simulink model "MVDR_example_hdl_4x4_systolic"  (R2020a)
settings: Solver=FixedStepDiscrete  StartTime=0.0  StopTime=stoptime  RelTol=1e-3
InitFcn:
  | model_init
values from neighbouring files (symbols this model uses):
  BackSubstitutePrototype = fi(0, matrixdivbacksub_dt)    [model_init.m]
  matrixDivDelay = NumberOfCORDICIterations*10 + 86    [model_init.m]
  movavg_bitshift = nextpow2(sqrt(windowSize))    [model_init.m]
  mvdrPipelineDelay = covMatDelay+movAvgDelay+matrixDivDelay+normResponseDelay    [model_init.m]
  numArrayElements = 4    [model_init.m]
  NumberOfCORDICIterations = matrixdivin_dt.WordLength - 1    [model_init.m]
  srcAngles = [20 60]    [model_init.m]
  sv = step(steeringVector,fc,[scanAngle; 0])    [model_init.m]
  Ts = 1/fs    (= 7.8125e-09)    [model_init.m]
  windowSize = 1024    [model_init.m]
libraries: hdlsllib x249, simulink x44, commfilt2 x4, commrfcorlib x3, commsync2 x3, commrflib2 x2, commrandsrc3 x2, phasedtxrxlib x2, commdigbbndcpm2 x1, dspsolvers x1, embreciprocals x1, commdigbbndpm3 x1
(part 4 of 11)

== system MVDR_example_hdl_4x4_systolic/MVDR HDL/Compute Weight Vector/Matrix Left Divide/CORDIC/4x4 Complex CORDIC Matrix Left Divide/Back Substitute 4x4 Complex CORDIC/Invert first element - Folded1/ValidIn to Ready Logic ==
  readyIn : Inport
  validIn : Inport  Port=2
  AND : Logic  IconShape=distinctive  AllPortsSameDT=off  OutDataTypeStr=boolean
  NOT : Logic  Operator=NOT  IconShape=distinctive  AllPortsSameDT=off  OutDataTypeStr=boolean
  readyOut : Outport  VectorParamsAs1DForOutWhenUnconnected=off
  wires:
  validIn/1 -> NOT/1
  readyIn/1 -> AND/1
  AND/1 -> readyOut/1
  NOT/1 -> AND/2

== system MVDR_example_hdl_4x4_systolic/MVDR HDL/Compute Weight Vector/Matrix Left Divide/CORDIC/4x4 Complex CORDIC Matrix Left Divide/Back Substitute 4x4 Complex CORDIC/Invert first element - Folded2/CORDIC Reciprocal Normalized, Folded ==
  x : Inport
  validIn : Inport  Port=2
  CORDIC Reciprocal Rotations- Folded : Subsystem  TreatAsAtomicUnit=on  mask{NumberOfCORDICIterations=NumberOfCORDICIterations}
      mask prompts: NumberOfCORDICIterations "Number of CORDIC Iterations"
  Change sign : MATLAB Function  TreatAsAtomicUnit=on
  Delay{,1..3,5,10} (6 alike) : Delay  DelayLength=1
  Normalizer : Subsystem
  State Control : StateControl  StateControl=Synchronous
  Unit Delay Enabled Synchronous : hdlsllib/Discrete/Unit Delay Enabled Synchronous  InitialCondition=0.0  SampleTime=-1
      settings: SourceProductBaseCode=SL
  Unit Delay Enabled Synchronous1 : hdlsllib/Discrete/Unit Delay Enabled Synchronous  InitialCondition=0.0  SampleTime=-1
      settings: SourceProductBaseCode=SL
  ValidIn to Ready Logic : Subsystem
  ValidIn to Ready Logic1 : Subsystem
  ValidIn to Ready Logic2 : Subsystem
  1/x_normalized : Outport  VectorParamsAs1DForOutWhenUnconnected=off
  shift_value : Outport  Port=2  VectorParamsAs1DForOutWhenUnconnected=off
  validOut : Outport  Port=3  VectorParamsAs1DForOutWhenUnconnected=off
  ready : Outport  Port=4  VectorParamsAs1DForOutWhenUnconnected=off
  wires:
  Delay1/1 -> ValidIn to Ready Logic/2(validIn), CORDIC Reciprocal Rotations- Folded/2(validIn)
  Delay2/1 -> validOut/1
  CORDIC Reciprocal Rotations- Folded/2(validOut) -> Delay2/1
  ValidIn to Ready Logic2/1(readyOut) -> ready/1
  ValidIn to Ready Logic1/1(readyOut) -> ValidIn to Ready Logic2/1(readyIn)
  ValidIn to Ready Logic/1(readyOut) -> ValidIn to Ready Logic1/1(readyIn)
  CORDIC Reciprocal Rotations- Folded/3(ready) -> ValidIn to Ready Logic/1(readyIn)
  Delay10/1 -> Normalizer/2(validIn), ValidIn to Ready Logic2/2(validIn)
  validIn/1 -> Delay10/1, Unit Delay Enabled Synchronous/2
  Normalizer/4(validOut) -> Unit Delay Enabled Synchronous1/2, Delay1/1, ValidIn to Ready Logic1/2(validIn)
  Delay/1 -> CORDIC Reciprocal Rotations- Folded/1(x_in)
  x/1 -> Unit Delay Enabled Synchronous/1
  Normalizer/3(shift_amount) -> Unit Delay Enabled Synchronous1/1
  CORDIC Reciprocal Rotations- Folded/1(z_out) -> Change sign/1(x)
  Delay5/1 -> shift_value/1
  Normalizer/2(is_negative) -> Change sign/2(is_negative)
  Delay3/1 -> 1/x_normalized/1
  Unit Delay Enabled Synchronous1/1 -> Delay5/1
  Change sign/1(y) -> Delay3/1
  Normalizer/1(u_normalized) -> Delay/1
  Unit Delay Enabled Synchronous/1 -> Normalizer/1(u)

== system MVDR_example_hdl_4x4_systolic/MVDR HDL/Compute Weight Vector/Matrix Left Divide/CORDIC/4x4 Complex CORDIC Matrix Left Divide/Back Substitute 4x4 Complex CORDIC/Invert first element - Folded2/ValidIn to Ready Logic ==
  readyIn : Inport
  validIn : Inport  Port=2
  AND : Logic  IconShape=distinctive  AllPortsSameDT=off  OutDataTypeStr=boolean
  NOT : Logic  Operator=NOT  IconShape=distinctive  AllPortsSameDT=off  OutDataTypeStr=boolean
  readyOut : Outport  VectorParamsAs1DForOutWhenUnconnected=off
  wires:
  validIn/1 -> NOT/1
  readyIn/1 -> AND/1
  AND/1 -> readyOut/1
  NOT/1 -> AND/2

== system MVDR_example_hdl_4x4_systolic/MVDR HDL/Compute Weight Vector/Matrix Left Divide/CORDIC/4x4 Complex CORDIC Matrix Left Divide/Back Substitute 4x4 Complex CORDIC/Invert first element - Folded3/CORDIC Reciprocal Normalized, Folded ==
  x : Inport
  validIn : Inport  Port=2
  CORDIC Reciprocal Rotations- Folded : Subsystem  TreatAsAtomicUnit=on  mask{NumberOfCORDICIterations=NumberOfCORDICIterations}
      mask prompts: NumberOfCORDICIterations "Number of CORDIC Iterations"
  Change sign : MATLAB Function  TreatAsAtomicUnit=on
  Delay{,1..3,5,10} (6 alike) : Delay  DelayLength=1
  Normalizer : Subsystem
  State Control : StateControl  StateControl=Synchronous
  Unit Delay Enabled Synchronous : hdlsllib/Discrete/Unit Delay Enabled Synchronous  InitialCondition=0.0  SampleTime=-1
      settings: SourceProductBaseCode=SL
  Unit Delay Enabled Synchronous1 : hdlsllib/Discrete/Unit Delay Enabled Synchronous  InitialCondition=0.0  SampleTime=-1
      settings: SourceProductBaseCode=SL
  ValidIn to Ready Logic : Subsystem
  ValidIn to Ready Logic1 : Subsystem
  ValidIn to Ready Logic2 : Subsystem
  1/x_normalized : Outport  VectorParamsAs1DForOutWhenUnconnected=off
  shift_value : Outport  Port=2  VectorParamsAs1DForOutWhenUnconnected=off
  validOut : Outport  Port=3  VectorParamsAs1DForOutWhenUnconnected=off
  ready : Outport  Port=4  VectorParamsAs1DForOutWhenUnconnected=off
  wires:
  Delay1/1 -> ValidIn to Ready Logic/2(validIn), CORDIC Reciprocal Rotations- Folded/2(validIn)
  Delay2/1 -> validOut/1
  CORDIC Reciprocal Rotations- Folded/2(validOut) -> Delay2/1
  ValidIn to Ready Logic2/1(readyOut) -> ready/1
  ValidIn to Ready Logic1/1(readyOut) -> ValidIn to Ready Logic2/1(readyIn)
  ValidIn to Ready Logic/1(readyOut) -> ValidIn to Ready Logic1/1(readyIn)
  CORDIC Reciprocal Rotations- Folded/3(ready) -> ValidIn to Ready Logic/1(readyIn)
  Delay10/1 -> Normalizer/2(validIn), ValidIn to Ready Logic2/2(validIn)
  validIn/1 -> Delay10/1, Unit Delay Enabled Synchronous/2
  Normalizer/4(validOut) -> Unit Delay Enabled Synchronous1/2, Delay1/1, ValidIn to Ready Logic1/2(validIn)
  Delay/1 -> CORDIC Reciprocal Rotations- Folded/1(x_in)
  x/1 -> Unit Delay Enabled Synchronous/1
  Normalizer/3(shift_amount) -> Unit Delay Enabled Synchronous1/1
  CORDIC Reciprocal Rotations- Folded/1(z_out) -> Change sign/1(x)
  Delay5/1 -> shift_value/1
  Normalizer/2(is_negative) -> Change sign/2(is_negative)
  Delay3/1 -> 1/x_normalized/1
  Unit Delay Enabled Synchronous1/1 -> Delay5/1
  Change sign/1(y) -> Delay3/1
  Normalizer/1(u_normalized) -> Delay/1
  Unit Delay Enabled Synchronous/1 -> Normalizer/1(u)

== system MVDR_example_hdl_4x4_systolic/MVDR HDL/Compute Weight Vector/Matrix Left Divide/CORDIC/4x4 Complex CORDIC Matrix Left Divide/Back Substitute 4x4 Complex CORDIC/Invert first element - Folded3/ValidIn to Ready Logic ==
  readyIn : Inport
  validIn : Inport  Port=2
  AND : Logic  IconShape=distinctive  AllPortsSameDT=off  OutDataTypeStr=boolean
  NOT : Logic  Operator=NOT  IconShape=distinctive  AllPortsSameDT=off  OutDataTypeStr=boolean
  readyOut : Outport  VectorParamsAs1DForOutWhenUnconnected=off
  wires:
  validIn/1 -> NOT/1
  readyIn/1 -> AND/1
  AND/1 -> readyOut/1
  NOT/1 -> AND/2

== system MVDR_example_hdl_4x4_systolic/MVDR HDL/Compute Weight Vector/Matrix Left Divide/CORDIC/4x4 Complex CORDIC Matrix Left Divide/Back Substitute 4x4 Complex CORDIC/Row1 Back Substitute Specify Output Type/Cast like prototype ==
  In1 : Inport
  Cast like output prototype : MATLAB Function  TreatAsAtomicUnit=on
  Out1 : Outport  VectorParamsAs1DForOutWhenUnconnected=off
  wires:
  In1/1 -> Cast like output prototype/1(x)
  Cast like output prototype/1(y) -> Out1/1

== system MVDR_example_hdl_4x4_systolic/MVDR HDL/Compute Weight Vector/Matrix Left Divide/CORDIC/4x4 Complex CORDIC Matrix Left Divide/Back Substitute 4x4 Complex CORDIC/Row1 Back Substitute Specify Output Type/Variable shift ==
  x : Inport
  shift_value : Inport  Port=2
  MATLAB Function : MATLAB Function  TreatAsAtomicUnit=on
  y : Outport  VectorParamsAs1DForOutWhenUnconnected=off
  wires:
  shift_value/1 -> MATLAB Function/2(shift_value)
  MATLAB Function/1(y) -> y/1
  x/1 -> MATLAB Function/1(x)

== system MVDR_example_hdl_4x4_systolic/MVDR HDL/Compute Weight Vector/Matrix Left Divide/CORDIC/4x4 Complex CORDIC Matrix Left Divide/Back Substitute 4x4 Complex CORDIC/Row1 Back Substitute Specify Output Type/x2*r1(2) ==
  note: Xilinx devices:
      | - Set D1 = 1-2, D4 = 1, D5 = 1
      | - Use sync reset
      |
      | Intel FPGAs:
      | - Set D1 = 1, D4 = 0, D5 = 1
      | - Use async reset
  In1 : Inport
  In2 : Inport  Port=2
  Add1 : Sum  Inputs=+-
  Add2 : Sum
  Complex to Real-Imag : ComplexToRealImag
  Complex to Real-Imag1 : ComplexToRealImag
  D1_1 : Delay  DelayLength=1
  D1_2 : Delay  DelayLength=1
  D4_{1..4} (4 alike) : Delay  DelayLength=1
  D5_1 : Delay  DelayLength=1
  D5_2 : Delay  DelayLength=1
  Product{1..4} (4 alike) : Product  OutDataTypeStr=Inherit: Same as first input
  Real-Imag to Complex : RealImagToComplex
  Out1 : Outport  VectorParamsAs1DForOutWhenUnconnected=off
  wires:
  D4_4/1 -> Add2/2
  D4_2/1 -> Add1/2
  Product4/1 -> D4_4/1
  D4_3/1 -> Add2/1
  Product2/1 -> D4_2/1
  D4_1/1 -> Add1/1
  D5_2/1 -> Real-Imag to Complex/2
  D5_1/1 -> Real-Imag to Complex/1
  Add2/1 -> D5_2/1
  Add1/1 -> D5_1/1
  Product3/1 -> D4_3/1
  Product1/1 -> D4_1/1
  Complex to Real-Imag1/2 -> Product2/2, Product4/2  "D"
  Complex to Real-Imag/2 -> Product2/1, Product3/1  "B"
  Complex to Real-Imag1/1 -> Product1/2, Product3/2  "C"
  Complex to Real-Imag/1 -> Product1/1, Product4/1  "A"
  D1_2/1 -> Complex to Real-Imag1/1
  D1_1/1 -> Complex to Real-Imag/1
  Real-Imag to Complex/1 -> Out1/1
  In1/1 -> D1_1/1
  In2/1 -> D1_2/1

== system MVDR_example_hdl_4x4_systolic/MVDR HDL/Compute Weight Vector/Matrix Left Divide/CORDIC/4x4 Complex CORDIC Matrix Left Divide/Back Substitute 4x4 Complex CORDIC/Row1 Back Substitute Specify Output Type/x3*r1(3) ==
  note: Xilinx devices:
      | - Set D1 = 1-2, D4 = 1, D5 = 1
      | - Use sync reset
      |
      | Intel FPGAs:
      | - Set D1 = 1, D4 = 0, D5 = 1
      | - Use async reset
  In1 : Inport
  In2 : Inport  Port=2
  Add1 : Sum  Inputs=+-
  Add2 : Sum
  Complex to Real-Imag : ComplexToRealImag
  Complex to Real-Imag1 : ComplexToRealImag
  D1_1 : Delay  DelayLength=1
  D1_2 : Delay  DelayLength=1
  D4_{1..4} (4 alike) : Delay  DelayLength=1
  D5_1 : Delay  DelayLength=1
  D5_2 : Delay  DelayLength=1
  Product{1..4} (4 alike) : Product  OutDataTypeStr=Inherit: Same as first input
  Real-Imag to Complex : RealImagToComplex
  Out1 : Outport  VectorParamsAs1DForOutWhenUnconnected=off
  wires:
  D4_4/1 -> Add2/2
  D4_2/1 -> Add1/2
  Product4/1 -> D4_4/1
  D4_3/1 -> Add2/1
  Product2/1 -> D4_2/1
  D4_1/1 -> Add1/1
  D5_2/1 -> Real-Imag to Complex/2
  D5_1/1 -> Real-Imag to Complex/1
  Add2/1 -> D5_2/1
  Add1/1 -> D5_1/1
  Product3/1 -> D4_3/1
  Product1/1 -> D4_1/1
  Complex to Real-Imag1/2 -> Product2/2, Product4/2  "D"
  Complex to Real-Imag/2 -> Product2/1, Product3/1  "B"
  Complex to Real-Imag1/1 -> Product1/2, Product3/2  "C"
  Complex to Real-Imag/1 -> Product1/1, Product4/1  "A"
  D1_2/1 -> Complex to Real-Imag1/1
  D1_1/1 -> Complex to Real-Imag/1
  Real-Imag to Complex/1 -> Out1/1
  In1/1 -> D1_1/1
  In2/1 -> D1_2/1

== system MVDR_example_hdl_4x4_systolic/MVDR HDL/Compute Weight Vector/Matrix Left Divide/CORDIC/4x4 Complex CORDIC Matrix Left Divide/Back Substitute 4x4 Complex CORDIC/Row1 Back Substitute Specify Output Type/x4*r1(4) ==
  note: Xilinx devices:
      | - Set D1 = 1-2, D4 = 1, D5 = 1
      | - Use sync reset
      |
      | Intel FPGAs:
      | - Set D1 = 1, D4 = 0, D5 = 1
      | - Use async reset
  In1 : Inport
  In2 : Inport  Port=2
  Add1 : Sum  Inputs=+-
  Add2 : Sum
  Complex to Real-Imag : ComplexToRealImag
  Complex to Real-Imag1 : ComplexToRealImag
  D1_1 : Delay  DelayLength=1
  D1_2 : Delay  DelayLength=1
  D4_{1..4} (4 alike) : Delay  DelayLength=1
  D5_1 : Delay  DelayLength=1
  D5_2 : Delay  DelayLength=1
  Product{1..4} (4 alike) : Product  OutDataTypeStr=Inherit: Same as first input
  Real-Imag to Complex : RealImagToComplex
  Out1 : Outport  VectorParamsAs1DForOutWhenUnconnected=off
  wires:
  D4_4/1 -> Add2/2
  D4_2/1 -> Add1/2
  Product4/1 -> D4_4/1
  D4_3/1 -> Add2/1
  Product2/1 -> D4_2/1
  D4_1/1 -> Add1/1
  D5_2/1 -> Real-Imag to Complex/2
  D5_1/1 -> Real-Imag to Complex/1
  Add2/1 -> D5_2/1
  Add1/1 -> D5_1/1
  Product3/1 -> D4_3/1
  Product1/1 -> D4_1/1
  Complex to Real-Imag1/2 -> Product2/2, Product4/2  "D"
  Complex to Real-Imag/2 -> Product2/1, Product3/1  "B"
  Complex to Real-Imag1/1 -> Product1/2, Product3/2  "C"
  Complex to Real-Imag/1 -> Product1/1, Product4/1  "A"
  D1_2/1 -> Complex to Real-Imag1/1
  D1_1/1 -> Complex to Real-Imag/1
  Real-Imag to Complex/1 -> Out1/1
  In1/1 -> D1_1/1
  In2/1 -> D1_2/1

== system MVDR_example_hdl_4x4_systolic/MVDR HDL/Compute Weight Vector/Matrix Left Divide/CORDIC/4x4 Complex CORDIC Matrix Left Divide/Back Substitute 4x4 Complex CORDIC/Row2 Back Substitute Specify Output Type/Cast like prototype ==
  In1 : Inport
  Cast like output prototype : MATLAB Function  TreatAsAtomicUnit=on
  Out1 : Outport  VectorParamsAs1DForOutWhenUnconnected=off
  wires:
  In1/1 -> Cast like output prototype/1(x)
  Cast like output prototype/1(y) -> Out1/1

== system MVDR_example_hdl_4x4_systolic/MVDR HDL/Compute Weight Vector/Matrix Left Divide/CORDIC/4x4 Complex CORDIC Matrix Left Divide/Back Substitute 4x4 Complex CORDIC/Row2 Back Substitute Specify Output Type/Variable shift ==
  x : Inport
  shift_value : Inport  Port=2
  MATLAB Function : MATLAB Function  TreatAsAtomicUnit=on
  y : Outport  VectorParamsAs1DForOutWhenUnconnected=off
  wires:
  shift_value/1 -> MATLAB Function/2(shift_value)
  MATLAB Function/1(y) -> y/1
  x/1 -> MATLAB Function/1(x)

== system MVDR_example_hdl_4x4_systolic/MVDR HDL/Compute Weight Vector/Matrix Left Divide/CORDIC/4x4 Complex CORDIC Matrix Left Divide/Back Substitute 4x4 Complex CORDIC/Row2 Back Substitute Specify Output Type/x3*r2(2) ==
  note: Xilinx devices:
      | - Set D1 = 1-2, D4 = 1, D5 = 1
      | - Use sync reset
      |
      | Intel FPGAs:
      | - Set D1 = 1, D4 = 0, D5 = 1
      | - Use async reset
  In1 : Inport
  In2 : Inport  Port=2
  Add1 : Sum  Inputs=+-
  Add2 : Sum
  Complex to Real-Imag : ComplexToRealImag
  Complex to Real-Imag1 : ComplexToRealImag
  D1_1 : Delay  DelayLength=1
  D1_2 : Delay  DelayLength=1
  D4_{1..4} (4 alike) : Delay  DelayLength=1
  D5_1 : Delay  DelayLength=1
  D5_2 : Delay  DelayLength=1
  Product{1..4} (4 alike) : Product  OutDataTypeStr=Inherit: Same as first input
  Real-Imag to Complex : RealImagToComplex
  Out1 : Outport  VectorParamsAs1DForOutWhenUnconnected=off
  wires:
  D4_4/1 -> Add2/2
  D4_2/1 -> Add1/2
  Product4/1 -> D4_4/1
  D4_3/1 -> Add2/1
  Product2/1 -> D4_2/1
  D4_1/1 -> Add1/1
  D5_2/1 -> Real-Imag to Complex/2
  D5_1/1 -> Real-Imag to Complex/1
  Add2/1 -> D5_2/1
  Add1/1 -> D5_1/1
  Product3/1 -> D4_3/1
  Product1/1 -> D4_1/1
  Complex to Real-Imag1/2 -> Product2/2, Product4/2  "D"
  Complex to Real-Imag/2 -> Product2/1, Product3/1  "B"
  Complex to Real-Imag1/1 -> Product1/2, Product3/2  "C"
  Complex to Real-Imag/1 -> Product1/1, Product4/1  "A"
  D1_2/1 -> Complex to Real-Imag1/1
  D1_1/1 -> Complex to Real-Imag/1
  Real-Imag to Complex/1 -> Out1/1
  In1/1 -> D1_1/1
  In2/1 -> D1_2/1

== system MVDR_example_hdl_4x4_systolic/MVDR HDL/Compute Weight Vector/Matrix Left Divide/CORDIC/4x4 Complex CORDIC Matrix Left Divide/Back Substitute 4x4 Complex CORDIC/Row2 Back Substitute Specify Output Type/x4*r2(3) ==
  note: Xilinx devices:
      | - Set D1 = 1-2, D4 = 1, D5 = 1
      | - Use sync reset
      |
      | Intel FPGAs:
      | - Set D1 = 1, D4 = 0, D5 = 1
      | - Use async reset
  In1 : Inport
  In2 : Inport  Port=2
  Add1 : Sum  Inputs=+-
  Add2 : Sum
  Complex to Real-Imag : ComplexToRealImag
  Complex to Real-Imag1 : ComplexToRealImag
  D1_1 : Delay  DelayLength=1
  D1_2 : Delay  DelayLength=1
  D4_{1..4} (4 alike) : Delay  DelayLength=1
  D5_1 : Delay  DelayLength=1
  D5_2 : Delay  DelayLength=1
  Product{1..4} (4 alike) : Product  OutDataTypeStr=Inherit: Same as first input
  Real-Imag to Complex : RealImagToComplex
  Out1 : Outport  VectorParamsAs1DForOutWhenUnconnected=off
  wires:
  D4_4/1 -> Add2/2
  D4_2/1 -> Add1/2
  Product4/1 -> D4_4/1
  D4_3/1 -> Add2/1
  Product2/1 -> D4_2/1
  D4_1/1 -> Add1/1
  D5_2/1 -> Real-Imag to Complex/2
  D5_1/1 -> Real-Imag to Complex/1
  Add2/1 -> D5_2/1
  Add1/1 -> D5_1/1
  Product3/1 -> D4_3/1
  Product1/1 -> D4_1/1
  Complex to Real-Imag1/2 -> Product2/2, Product4/2  "D"
  Complex to Real-Imag/2 -> Product2/1, Product3/1  "B"
  Complex to Real-Imag1/1 -> Product1/2, Product3/2  "C"
  Complex to Real-Imag/1 -> Product1/1, Product4/1  "A"
  D1_2/1 -> Complex to Real-Imag1/1
  D1_1/1 -> Complex to Real-Imag/1
  Real-Imag to Complex/1 -> Out1/1
  In1/1 -> D1_1/1
  In2/1 -> D1_2/1

== system MVDR_example_hdl_4x4_systolic/MVDR HDL/Compute Weight Vector/Matrix Left Divide/CORDIC/4x4 Complex CORDIC Matrix Left Divide/Back Substitute 4x4 Complex CORDIC/Row3 Back Substitute Specify Output Type/Cast like prototype ==
  In1 : Inport
  Cast like output prototype : MATLAB Function  TreatAsAtomicUnit=on
  Out1 : Outport  VectorParamsAs1DForOutWhenUnconnected=off
  wires:
  In1/1 -> Cast like output prototype/1(x)
  Cast like output prototype/1(y) -> Out1/1

== system MVDR_example_hdl_4x4_systolic/MVDR HDL/Compute Weight Vector/Matrix Left Divide/CORDIC/4x4 Complex CORDIC Matrix Left Divide/Back Substitute 4x4 Complex CORDIC/Row3 Back Substitute Specify Output Type/Cast like prototype1 ==
  In1 : Inport
  Cast like output prototype : MATLAB Function  TreatAsAtomicUnit=on
  Out1 : Outport  VectorParamsAs1DForOutWhenUnconnected=off
  wires:
  In1/1 -> Cast like output prototype/1(x)
  Cast like output prototype/1(y) -> Out1/1

== system MVDR_example_hdl_4x4_systolic/MVDR HDL/Compute Weight Vector/Matrix Left Divide/CORDIC/4x4 Complex CORDIC Matrix Left Divide/Back Substitute 4x4 Complex CORDIC/Row3 Back Substitute Specify Output Type/Variable shift ==
  x : Inport
  shift_value : Inport  Port=2
  MATLAB Function : MATLAB Function  TreatAsAtomicUnit=on
  y : Outport  VectorParamsAs1DForOutWhenUnconnected=off
  wires:
  shift_value/1 -> MATLAB Function/2(shift_value)
  MATLAB Function/1(y) -> y/1
  x/1 -> MATLAB Function/1(x)

== system MVDR_example_hdl_4x4_systolic/MVDR HDL/Compute Weight Vector/Matrix Left Divide/CORDIC/4x4 Complex CORDIC Matrix Left Divide/Back Substitute 4x4 Complex CORDIC/Row3 Back Substitute Specify Output Type/r3(2)*x4 ==
  note: Xilinx devices:
      | - Set D1 = 1-2, D4 = 1, D5 = 1
      | - Use sync reset
      |
      | Intel FPGAs:
      | - Set D1 = 1, D4 = 0, D5 = 1
      | - Use async reset
  In1 : Inport
  In2 : Inport  Port=2
  Add1 : Sum  Inputs=+-
  Add2 : Sum
  Complex to Real-Imag : ComplexToRealImag
  Complex to Real-Imag1 : ComplexToRealImag
  D1_1 : Delay  DelayLength=1
  D1_2 : Delay  DelayLength=1
  D4_{1..4} (4 alike) : Delay  DelayLength=1
  D5_1 : Delay  DelayLength=1
  D5_2 : Delay  DelayLength=1
  Product{1..4} (4 alike) : Product  OutDataTypeStr=Inherit: Same as first input
  Real-Imag to Complex : RealImagToComplex
  Out1 : Outport  VectorParamsAs1DForOutWhenUnconnected=off
  wires:
  D4_4/1 -> Add2/2
  D4_2/1 -> Add1/2
  Product4/1 -> D4_4/1
  D4_3/1 -> Add2/1
  Product2/1 -> D4_2/1
  D4_1/1 -> Add1/1
  D5_2/1 -> Real-Imag to Complex/2
  D5_1/1 -> Real-Imag to Complex/1
  Add2/1 -> D5_2/1
  Add1/1 -> D5_1/1
  Product3/1 -> D4_3/1
  Product1/1 -> D4_1/1
  Complex to Real-Imag1/2 -> Product2/2, Product4/2  "D"
  Complex to Real-Imag/2 -> Product2/1, Product3/1  "B"
  Complex to Real-Imag1/1 -> Product1/2, Product3/2  "C"
  Complex to Real-Imag/1 -> Product1/1, Product4/1  "A"
  D1_2/1 -> Complex to Real-Imag1/1
  D1_1/1 -> Complex to Real-Imag/1
  Real-Imag to Complex/1 -> Out1/1
  In1/1 -> D1_1/1
  In2/1 -> D1_2/1

== system MVDR_example_hdl_4x4_systolic/MVDR HDL/Compute Weight Vector/Matrix Left Divide/CORDIC/4x4 Complex CORDIC Matrix Left Divide/Back Substitute 4x4 Complex CORDIC/Row4 Back Substitute Specify Output Type/Cast like prototype ==
  In1 : Inport
  Cast like output prototype : MATLAB Function  TreatAsAtomicUnit=on
  Out1 : Outport  VectorParamsAs1DForOutWhenUnconnected=off
  wires:
  In1/1 -> Cast like output prototype/1(x)
  Cast like output prototype/1(y) -> Out1/1

== system MVDR_example_hdl_4x4_systolic/MVDR HDL/Compute Weight Vector/Matrix Left Divide/CORDIC/4x4 Complex CORDIC Matrix Left Divide/Back Substitute 4x4 Complex CORDIC/Row4 Back Substitute Specify Output Type/Variable shift ==
  x : Inport
  shift_value : Inport  Port=2
  MATLAB Function : MATLAB Function  TreatAsAtomicUnit=on
  y : Outport  VectorParamsAs1DForOutWhenUnconnected=off
  wires:
  shift_value/1 -> MATLAB Function/2(shift_value)
  MATLAB Function/1(y) -> y/1
  x/1 -> MATLAB Function/1(x)

== system MVDR_example_hdl_4x4_systolic/MVDR HDL/Compute Weight Vector/Matrix Left Divide/CORDIC/4x4 Complex CORDIC Matrix Left Divide/Q'B, R 4x4 Complex CORDIC Systolic Array/Complex Row Rotation with real pivots/Inverse CORDIC Gain1 ==
  In1 : Inport
  Inverse CORDIC Gain : Gain  Gain=1/prod(sqrt(1+2.^(-2*(0:double(NumberOfCORDICIterations)-1))))  OutDataTypeStr=Inherit: Same as input
  Out1 : Outport  VectorParamsAs1DForOutWhenUnconnected=off
  wires:
  Inverse CORDIC Gain/1 -> Out1/1
  In1/1 -> Inverse CORDIC Gain/1

== system MVDR_example_hdl_4x4_systolic/MVDR HDL/Compute Weight Vector/Matrix Left Divide/CORDIC/4x4 Complex CORDIC Matrix Left Divide/Q'B, R 4x4 Complex CORDIC Systolic Array/Complex Row Rotation with real pivots/Inverse CORDIC Gain2 ==
  In1 : Inport
  Inverse CORDIC Gain : Gain  Gain=1/prod(sqrt(1+2.^(-2*(0:double(NumberOfCORDICIterations)-1))))  OutDataTypeStr=Inherit: Same as input
  Out1 : Outport  VectorParamsAs1DForOutWhenUnconnected=off
  wires:
  Inverse CORDIC Gain/1 -> Out1/1
  In1/1 -> Inverse CORDIC Gain/1

== system MVDR_example_hdl_4x4_systolic/MVDR HDL/Compute Weight Vector/Matrix Left Divide/CORDIC/4x4 Complex CORDIC Matrix Left Divide/Q'B, R 4x4 Complex CORDIC Systolic Array/Complex Row Rotation with real pivots/Inverse CORDIC Gain3 ==
  In1 : Inport
  Inverse CORDIC Gain : Gain  Gain=1/prod(sqrt(1+2.^(-2*(0:double(NumberOfCORDICIterations)-1))))  OutDataTypeStr=Inherit: Same as input
  Out1 : Outport  VectorParamsAs1DForOutWhenUnconnected=off
  wires:
  Inverse CORDIC Gain/1 -> Out1/1
  In1/1 -> Inverse CORDIC Gain/1

== system MVDR_example_hdl_4x4_systolic/MVDR HDL/Compute Weight Vector/Matrix Left Divide/CORDIC/4x4 Complex CORDIC Matrix Left Divide/Q'B, R 4x4 Complex CORDIC Systolic Array/Complex Row Rotation with real pivots/Inverse CORDIC Gain4 ==
  In1 : Inport
  Inverse CORDIC Gain : Gain  Gain=1/prod(sqrt(1+2.^(-2*(0:double(NumberOfCORDICIterations)-1))))  OutDataTypeStr=Inherit: Same as input
  Out1 : Outport  VectorParamsAs1DForOutWhenUnconnected=off
  wires:
  Inverse CORDIC Gain/1 -> Out1/1
  In1/1 -> Inverse CORDIC Gain/1

== system MVDR_example_hdl_4x4_systolic/MVDR HDL/Compute Weight Vector/Matrix Left Divide/CORDIC/4x4 Complex CORDIC Matrix Left Divide/Q'B, R 4x4 Complex CORDIC Systolic Array/Complex Row Rotation with real pivots/Q'B, R Row Rotations - Complex ==
  x : Inport
  y : Inport  Port=2
  u : Inport  Port=3
  v : Inport  Port=4
  validIn : Inport  Port=5
  CORDIC Counter : Subsystem  mask{NumberOfCORDICIterations=NumberOfCORDICIterations}
      mask prompts: NumberOfCORDICIterations "Number of CORDIC Iterations"
  Delay{1..13} (13 alike) : Delay  DelayLength=1
  MATLAB Function : MATLAB Function  TreatAsAtomicUnit=on
  Same Datatype : Subsystem  TreatAsAtomicUnit=on
  Same Datatype1 : Subsystem  TreatAsAtomicUnit=on
  Same Datatype2 : Subsystem  TreatAsAtomicUnit=on
  Same Datatype3 : Subsystem  TreatAsAtomicUnit=on
  Switch{,1..3} (4 alike) : Switch  Criteria=u2 ~= 0
  x_out : Outport  VectorParamsAs1DForOutWhenUnconnected=off
  y_out : Outport  Port=2  VectorParamsAs1DForOutWhenUnconnected=off
  u_out : Outport  Port=3  VectorParamsAs1DForOutWhenUnconnected=off
  v_out : Outport  Port=4  VectorParamsAs1DForOutWhenUnconnected=off
  validOut : Outport  Port=5  VectorParamsAs1DForOutWhenUnconnected=off
  ready : Outport  Port=6  VectorParamsAs1DForOutWhenUnconnected=off
  wires:
  Delay13/1 -> ready/1
  Delay12/1 -> Delay3/1
  Delay10/1 -> MATLAB Function/5(iteration)
  Delay9/1 -> Switch3/2, Switch2/2, Switch1/2, Switch/2
  Delay8/1 -> Switch3/3, Same Datatype2/2(Reference)
  Delay6/1 -> Switch2/3, Same Datatype3/2(Reference)
  Delay5/1 -> Switch1/3, Same Datatype1/2(Reference)
  Delay4/1 -> Switch/3, Same Datatype/2(Reference)
  Same Datatype2/1(DataOut) -> Switch3/1
  Same Datatype3/1(DataOut) -> Switch2/1
  Same Datatype1/1(DataOut) -> Switch1/1
  Same Datatype/1(DataOut) -> Switch/1
  v/1 -> Delay8/1
  u/1 -> Delay6/1
  y/1 -> Delay5/1
  x/1 -> Delay4/1
  CORDIC Counter/1(count_is_positive) -> Delay9/1
  Switch3/1 -> MATLAB Function/4(v)
  Switch2/1 -> MATLAB Function/3(u)
  Switch1/1 -> MATLAB Function/2(y)
  Switch/1 -> MATLAB Function/1(x)
  CORDIC Counter/4(ready) -> Delay13/1
  CORDIC Counter/3(last) -> Delay12/1
  CORDIC Counter/2(count) -> Delay10/1
  validIn/1 -> CORDIC Counter/1(validIn)
  Delay3/1 -> validOut/1
  Delay7/1 -> u_out/1, Same Datatype3/1(Data)
  MATLAB Function/4(v_out) -> Delay11/1
  MATLAB Function/3(u_out) -> Delay7/1
  MATLAB Function/2(y_out) -> Delay2/1
  MATLAB Function/1(x_out) -> Delay1/1
  Delay11/1 -> v_out/1, Same Datatype2/1(Data)
  Delay2/1 -> y_out/1, Same Datatype1/1(Data)
  Delay1/1 -> x_out/1, Same Datatype/1(Data)

== system MVDR_example_hdl_4x4_systolic/MVDR HDL/Compute Weight Vector/Matrix Left Divide/CORDIC/4x4 Complex CORDIC Matrix Left Divide/Q'B, R 4x4 Complex CORDIC Systolic Array/Complex Row Rotation with real pivots/ValidIn to Ready Logic ==
  readyIn : Inport
  validIn : Inport  Port=2
  AND : Logic  IconShape=distinctive  AllPortsSameDT=off  OutDataTypeStr=boolean
  NOT : Logic  Operator=NOT  IconShape=distinctive  AllPortsSameDT=off  OutDataTypeStr=boolean
  readyOut : Outport  VectorParamsAs1DForOutWhenUnconnected=off
  wires:
  validIn/1 -> NOT/1
  readyIn/1 -> AND/1
  AND/1 -> readyOut/1
  NOT/1 -> AND/2

== system MVDR_example_hdl_4x4_systolic/MVDR HDL/Compute Weight Vector/Matrix Left Divide/CORDIC/4x4 Complex CORDIC Matrix Left Divide/Q'B, R 4x4 Complex CORDIC Systolic Array/Complex Row Rotation with real pivots/ValidIn to Ready Logic1 ==
  readyIn : Inport
  validIn : Inport  Port=2
  AND : Logic  IconShape=distinctive  AllPortsSameDT=off  OutDataTypeStr=boolean
  NOT : Logic  Operator=NOT  IconShape=distinctive  AllPortsSameDT=off  OutDataTypeStr=boolean
  readyOut : Outport  VectorParamsAs1DForOutWhenUnconnected=off
  wires:
  validIn/1 -> NOT/1
  readyIn/1 -> AND/1
  AND/1 -> readyOut/1
  NOT/1 -> AND/2

== system MVDR_example_hdl_4x4_systolic/MVDR HDL/Compute Weight Vector/Matrix Left Divide/CORDIC/4x4 Complex CORDIC Matrix Left Divide/Q'B, R 4x4 Complex CORDIC Systolic Array/Complex Row Rotation 1/Inverse CORDIC Gain1 ==
  In1 : Inport
  Inverse CORDIC Gain : Gain  Gain=1/prod(sqrt(1+2.^(-2*(0:double(NumberOfCORDICIterations)-1))))  OutDataTypeStr=Inherit: Same as input
  Out1 : Outport  VectorParamsAs1DForOutWhenUnconnected=off
  wires:
  Inverse CORDIC Gain/1 -> Out1/1
  In1/1 -> Inverse CORDIC Gain/1

== system MVDR_example_hdl_4x4_systolic/MVDR HDL/Compute Weight Vector/Matrix Left Divide/CORDIC/4x4 Complex CORDIC Matrix Left Divide/Q'B, R 4x4 Complex CORDIC Systolic Array/Complex Row Rotation 1/Inverse CORDIC Gain2 ==
  In1 : Inport
  Inverse CORDIC Gain : Gain  Gain=1/prod(sqrt(1+2.^(-2*(0:double(NumberOfCORDICIterations)-1))))  OutDataTypeStr=Inherit: Same as input
  Out1 : Outport  VectorParamsAs1DForOutWhenUnconnected=off
  wires:
  Inverse CORDIC Gain/1 -> Out1/1
  In1/1 -> Inverse CORDIC Gain/1

== system MVDR_example_hdl_4x4_systolic/MVDR HDL/Compute Weight Vector/Matrix Left Divide/CORDIC/4x4 Complex CORDIC Matrix Left Divide/Q'B, R 4x4 Complex CORDIC Systolic Array/Complex Row Rotation 1/Inverse CORDIC Gain3 ==
  In1 : Inport
  Inverse CORDIC Gain : Gain  Gain=1/prod(sqrt(1+2.^(-2*(0:double(NumberOfCORDICIterations)-1))))  OutDataTypeStr=Inherit: Same as input
  Out1 : Outport  VectorParamsAs1DForOutWhenUnconnected=off
  wires:
  Inverse CORDIC Gain/1 -> Out1/1
  In1/1 -> Inverse CORDIC Gain/1

== system MVDR_example_hdl_4x4_systolic/MVDR HDL/Compute Weight Vector/Matrix Left Divide/CORDIC/4x4 Complex CORDIC Matrix Left Divide/Q'B, R 4x4 Complex CORDIC Systolic Array/Complex Row Rotation 1/Inverse CORDIC Gain4 ==
  In1 : Inport
  Inverse CORDIC Gain : Gain  Gain=1/prod(sqrt(1+2.^(-2*(0:double(NumberOfCORDICIterations)-1))))  OutDataTypeStr=Inherit: Same as input
  Out1 : Outport  VectorParamsAs1DForOutWhenUnconnected=off
  wires:
  Inverse CORDIC Gain/1 -> Out1/1
  In1/1 -> Inverse CORDIC Gain/1

== system MVDR_example_hdl_4x4_systolic/MVDR HDL/Compute Weight Vector/Matrix Left Divide/CORDIC/4x4 Complex CORDIC Matrix Left Divide/Q'B, R 4x4 Complex CORDIC Systolic Array/Complex Row Rotation 1/Q'B, R Row Rotations - Complex - Folded ==
  x : Inport
  y : Inport  Port=2
  u : Inport  Port=3
  v : Inport  Port=4
  validIn : Inport  Port=5
  CORDIC Counter : Subsystem  mask{NumberOfCORDICIterations=NumberOfCORDICIterations}
      mask prompts: NumberOfCORDICIterations "Number of CORDIC Iterations"
  Delay{1..13} (13 alike) : Delay  DelayLength=1
  MATLAB Function : MATLAB Function  TreatAsAtomicUnit=on
  Same Datatype : Subsystem  TreatAsAtomicUnit=on
  Same Datatype1 : Subsystem  TreatAsAtomicUnit=on
  Same Datatype2 : Subsystem  TreatAsAtomicUnit=on
  Same Datatype3 : Subsystem  TreatAsAtomicUnit=on
  Switch{,1..3} (4 alike) : Switch  Criteria=u2 ~= 0
  x_out : Outport  VectorParamsAs1DForOutWhenUnconnected=off
  y_out : Outport  Port=2  VectorParamsAs1DForOutWhenUnconnected=off
  u_out : Outport  Port=3  VectorParamsAs1DForOutWhenUnconnected=off
  v_out : Outport  Port=4  VectorParamsAs1DForOutWhenUnconnected=off
  validOut : Outport  Port=5  VectorParamsAs1DForOutWhenUnconnected=off
  ready : Outport  Port=6  VectorParamsAs1DForOutWhenUnconnected=off
  wires:
  Delay13/1 -> ready/1
  Delay12/1 -> Delay3/1
  Delay10/1 -> MATLAB Function/5(iteration)
  Delay9/1 -> Switch3/2, Switch2/2, Switch1/2, Switch/2
  Delay8/1 -> Switch3/3, Same Datatype2/2(Reference)
  Delay6/1 -> Switch2/3, Same Datatype3/2(Reference)
  Delay5/1 -> Switch1/3, Same Datatype1/2(Reference)
  Delay4/1 -> Switch/3, Same Datatype/2(Reference)
  Same Datatype2/1(DataOut) -> Switch3/1
  Same Datatype3/1(DataOut) -> Switch2/1
  Same Datatype1/1(DataOut) -> Switch1/1
  Same Datatype/1(DataOut) -> Switch/1
  v/1 -> Delay8/1
  u/1 -> Delay6/1
  y/1 -> Delay5/1
  x/1 -> Delay4/1
  CORDIC Counter/1(count_is_positive) -> Delay9/1
  Switch3/1 -> MATLAB Function/4(v)
  Switch2/1 -> MATLAB Function/3(u)
  Switch1/1 -> MATLAB Function/2(y)
  Switch/1 -> MATLAB Function/1(x)
  CORDIC Counter/4(ready) -> Delay13/1
  CORDIC Counter/3(last) -> Delay12/1
  CORDIC Counter/2(count) -> Delay10/1
  validIn/1 -> CORDIC Counter/1(validIn)
  Delay3/1 -> validOut/1
  Delay7/1 -> u_out/1, Same Datatype3/1(Data)
  MATLAB Function/4(v_out) -> Delay11/1
  MATLAB Function/3(u_out) -> Delay7/1
  MATLAB Function/2(y_out) -> Delay2/1
  MATLAB Function/1(x_out) -> Delay1/1
  Delay11/1 -> v_out/1, Same Datatype2/1(Data)
  Delay2/1 -> y_out/1, Same Datatype1/1(Data)
  Delay1/1 -> x_out/1, Same Datatype/1(Data)

== system MVDR_example_hdl_4x4_systolic/MVDR HDL/Compute Weight Vector/Matrix Left Divide/CORDIC/4x4 Complex CORDIC Matrix Left Divide/Q'B, R 4x4 Complex CORDIC Systolic Array/Complex Row Rotation 1/Rotate first element to real - Folded ==
  x : Inport
  u : Inport  Port=2
  validIn : Inport  Port=3
  Complex to Real-Imag : ComplexToRealImag
  Complex to Real-Imag1 : ComplexToRealImag
  Delay{4..7,9..10,15} (7 alike) : Delay  DelayLength=1
  Force imaginary part to exactly zero : MATLAB Function  TreatAsAtomicUnit=on
  Inverse CORDIC Gain1 : Subsystem  TreatAsAtomicUnit=on  mask{NumberOfCORDICIterations=NumberOfCORDICIterations}
      mask prompts: NumberOfCORDICIterations "Number of CORDIC Iterations"
      mask Display: disp('1/An')
  Inverse CORDIC Gain2 : Subsystem  TreatAsAtomicUnit=on  mask{NumberOfCORDICIterations=NumberOfCORDICIterations}
      mask prompts: NumberOfCORDICIterations "Number of CORDIC Iterations"
      mask Display: disp('1/An')
  Inverse CORDIC Gain3 : Subsystem  TreatAsAtomicUnit=on  mask{NumberOfCORDICIterations=NumberOfCORDICIterations}
      mask prompts: NumberOfCORDICIterations "Number of CORDIC Iterations"
      mask Display: disp('1/An')
  Inverse CORDIC Gain4 : Subsystem  TreatAsAtomicUnit=on  mask{NumberOfCORDICIterations=NumberOfCORDICIterations}
      mask prompts: NumberOfCORDICIterations "Number of CORDIC Iterations"
      mask Display: disp('1/An')
  "Q'B, R Row Rotations - Real" : Subsystem  TreatAsAtomicUnit=on  mask{NumberOfCORDICIterations=NumberOfCORDICIterations}
      mask prompts: NumberOfCORDICIterations "Number of CORDIC Iterations"
  QR 3rd and 4th Quadrant Compensation : MATLAB Function  TreatAsAtomicUnit=on
  Real-Imag to Complex : RealImagToComplex
  Real-Imag to Complex1 : RealImagToComplex
  State Control : StateControl  StateControl=Synchronous
  Unit Delay Enabled Synchronous{,1..3} (4 alike) : hdlsllib/Discrete/Unit Delay Enabled Synchronous  InitialCondition=0.0  SampleTime=-1
      settings: SourceProductBaseCode=SL
  ValidIn to Ready Logic with Delay : Subsystem
  x' : Outport  VectorParamsAs1DForOutWhenUnconnected=off
  u' : Outport  Port=2  VectorParamsAs1DForOutWhenUnconnected=off
  validOut : Outport  Port=3  VectorParamsAs1DForOutWhenUnconnected=off
  ready : Outport  Port=4  VectorParamsAs1DForOutWhenUnconnected=off
  wires:
  Unit Delay Enabled Synchronous3/1 -> x'/1
  Real-Imag to Complex/1 -> Unit Delay Enabled Synchronous3/1
  Unit Delay Enabled Synchronous2/1 -> u'/1
  Real-Imag to Complex1/1 -> Unit Delay Enabled Synchronous2/1
  Unit Delay Enabled Synchronous1/1 -> Complex to Real-Imag/1
  Unit Delay Enabled Synchronous/1 -> Complex to Real-Imag1/1
  "Q'B, R Row Rotations - Real"/6(ready) -> ValidIn to Ready Logic with Delay/1(readyIn)
  ValidIn to Ready Logic with Delay/1(readyOut) -> ready/1
  Delay15/1 -> validOut/1
  "Q'B, R Row Rotations - Real"/5(validOut) -> Delay15/1, Unit Delay Enabled Synchronous3/2, Unit Delay Enabled Synchronous2/2
  Inverse CORDIC Gain3/1(Out1) -> Real-Imag to Complex1/2
  Inverse CORDIC Gain2/1(Out1) -> Real-Imag to Complex1/1
  Inverse CORDIC Gain1/1(Out1) -> Force imaginary part to exactly zero/1(u)
  Inverse CORDIC Gain4/1(Out1) -> Real-Imag to Complex/1
  Delay10/1 -> "Q'B, R Row Rotations - Real"/5(validIn), ValidIn to Ready Logic with Delay/2(validIn * z^-1)
  validIn/1 -> Delay9/1, Unit Delay Enabled Synchronous1/2, Unit Delay Enabled Synchronous/2
  Delay9/1 -> Delay10/1, ValidIn to Ready Logic with Delay/3(validIn)
  Force imaginary part to exactly zero/1(y) -> Real-Imag to Complex/2
  "Q'B, R Row Rotations - Real"/2(y_out) -> Inverse CORDIC Gain1/1(In1)
  u/1 -> Unit Delay Enabled Synchronous/1
  x/1 -> Unit Delay Enabled Synchronous1/1
  "Q'B, R Row Rotations - Real"/4(v_out) -> Inverse CORDIC Gain3/1(In1)
  "Q'B, R Row Rotations - Real"/3(u_out) -> Inverse CORDIC Gain2/1(In1)
  "Q'B, R Row Rotations - Real"/1(x_out) -> Inverse CORDIC Gain4/1(In1)
  Delay7/1 -> "Q'B, R Row Rotations - Real"/4(v)
  Delay6/1 -> "Q'B, R Row Rotations - Real"/3(u)
  Delay5/1 -> "Q'B, R Row Rotations - Real"/2(y)
  Delay4/1 -> "Q'B, R Row Rotations - Real"/1(x)
  Complex to Real-Imag1/2 -> QR 3rd and 4th Quadrant Compensation/4(v)
  Complex to Real-Imag1/1 -> QR 3rd and 4th Quadrant Compensation/3(u)
  Complex to Real-Imag/2 -> QR 3rd and 4th Quadrant Compensation/2(y)
  Complex to Real-Imag/1 -> QR 3rd and 4th Quadrant Compensation/1(x)
  QR 3rd and 4th Quadrant Compensation/4(v_out) -> Delay7/1
  QR 3rd and 4th Quadrant Compensation/2(y_out) -> Delay5/1
  QR 3rd and 4th Quadrant Compensation/3(u_out) -> Delay6/1
  QR 3rd and 4th Quadrant Compensation/1(x_out) -> Delay4/1

== system MVDR_example_hdl_4x4_systolic/MVDR HDL/Compute Weight Vector/Matrix Left Divide/CORDIC/4x4 Complex CORDIC Matrix Left Divide/Q'B, R 4x4 Complex CORDIC Systolic Array/Complex Row Rotation 1/ValidIn to Ready Logic ==
  readyIn : Inport
  validIn : Inport  Port=2
  AND : Logic  IconShape=distinctive  AllPortsSameDT=off  OutDataTypeStr=boolean
  NOT : Logic  Operator=NOT  IconShape=distinctive  AllPortsSameDT=off  OutDataTypeStr=boolean
  readyOut : Outport  VectorParamsAs1DForOutWhenUnconnected=off
  wires:
  validIn/1 -> NOT/1
  readyIn/1 -> AND/1
  AND/1 -> readyOut/1
  NOT/1 -> AND/2

== system MVDR_example_hdl_4x4_systolic/MVDR HDL/Compute Weight Vector/Matrix Left Divide/CORDIC/4x4 Complex CORDIC Matrix Left Divide/Q'B, R 4x4 Complex CORDIC Systolic Array/Complex Row Rotation 1/ValidIn to Ready Logic1 ==
  readyIn : Inport
  validIn : Inport  Port=2
  AND : Logic  IconShape=distinctive  AllPortsSameDT=off  OutDataTypeStr=boolean
  NOT : Logic  Operator=NOT  IconShape=distinctive  AllPortsSameDT=off  OutDataTypeStr=boolean
  readyOut : Outport  VectorParamsAs1DForOutWhenUnconnected=off
  wires:
  validIn/1 -> NOT/1
  readyIn/1 -> AND/1
  AND/1 -> readyOut/1
  NOT/1 -> AND/2

== system MVDR_example_hdl_4x4_systolic/MVDR HDL/Compute Weight Vector/Matrix Left Divide/CORDIC/4x4 Complex CORDIC Matrix Left Divide/Q'B, R 4x4 Complex CORDIC Systolic Array/Leading Complex Row Rotation/Inverse CORDIC Gain1 ==
  In1 : Inport
  Inverse CORDIC Gain : Gain  Gain=1/prod(sqrt(1+2.^(-2*(0:double(NumberOfCORDICIterations)-1))))  OutDataTypeStr=Inherit: Same as input
  Out1 : Outport  VectorParamsAs1DForOutWhenUnconnected=off
  wires:
  Inverse CORDIC Gain/1 -> Out1/1
  In1/1 -> Inverse CORDIC Gain/1

== system MVDR_example_hdl_4x4_systolic/MVDR HDL/Compute Weight Vector/Matrix Left Divide/CORDIC/4x4 Complex CORDIC Matrix Left Divide/Q'B, R 4x4 Complex CORDIC Systolic Array/Leading Complex Row Rotation/Inverse CORDIC Gain2 ==
  In1 : Inport
  Inverse CORDIC Gain : Gain  Gain=1/prod(sqrt(1+2.^(-2*(0:double(NumberOfCORDICIterations)-1))))  OutDataTypeStr=Inherit: Same as input
  Out1 : Outport  VectorParamsAs1DForOutWhenUnconnected=off
  wires:
  Inverse CORDIC Gain/1 -> Out1/1
  In1/1 -> Inverse CORDIC Gain/1

== system MVDR_example_hdl_4x4_systolic/MVDR HDL/Compute Weight Vector/Matrix Left Divide/CORDIC/4x4 Complex CORDIC Matrix Left Divide/Q'B, R 4x4 Complex CORDIC Systolic Array/Leading Complex Row Rotation/Inverse CORDIC Gain3 ==
  In1 : Inport
  Inverse CORDIC Gain : Gain  Gain=1/prod(sqrt(1+2.^(-2*(0:double(NumberOfCORDICIterations)-1))))  OutDataTypeStr=Inherit: Same as input
  Out1 : Outport  VectorParamsAs1DForOutWhenUnconnected=off
  wires:
  Inverse CORDIC Gain/1 -> Out1/1
  In1/1 -> Inverse CORDIC Gain/1

== system MVDR_example_hdl_4x4_systolic/MVDR HDL/Compute Weight Vector/Matrix Left Divide/CORDIC/4x4 Complex CORDIC Matrix Left Divide/Q'B, R 4x4 Complex CORDIC Systolic Array/Leading Complex Row Rotation/Inverse CORDIC Gain4 ==
  In1 : Inport
  Inverse CORDIC Gain : Gain  Gain=1/prod(sqrt(1+2.^(-2*(0:double(NumberOfCORDICIterations)-1))))  OutDataTypeStr=Inherit: Same as input
  Out1 : Outport  VectorParamsAs1DForOutWhenUnconnected=off
  wires:
  Inverse CORDIC Gain/1 -> Out1/1
  In1/1 -> Inverse CORDIC Gain/1

== system MVDR_example_hdl_4x4_systolic/MVDR HDL/Compute Weight Vector/Matrix Left Divide/CORDIC/4x4 Complex CORDIC Matrix Left Divide/Q'B, R 4x4 Complex CORDIC Systolic Array/Leading Complex Row Rotation/Q'B, R Row Rotations - Complex ==
  x : Inport
  y : Inport  Port=2
  u : Inport  Port=3
  v : Inport  Port=4
  validIn : Inport  Port=5
  CORDIC Counter : Subsystem  mask{NumberOfCORDICIterations=NumberOfCORDICIterations}
      mask prompts: NumberOfCORDICIterations "Number of CORDIC Iterations"
  Delay{1..13} (13 alike) : Delay  DelayLength=1
  MATLAB Function : MATLAB Function  TreatAsAtomicUnit=on
  Same Datatype : Subsystem  TreatAsAtomicUnit=on
  Same Datatype1 : Subsystem  TreatAsAtomicUnit=on
  Same Datatype2 : Subsystem  TreatAsAtomicUnit=on
  Same Datatype3 : Subsystem  TreatAsAtomicUnit=on
  Switch{,1..3} (4 alike) : Switch  Criteria=u2 ~= 0
  x_out : Outport  VectorParamsAs1DForOutWhenUnconnected=off
  y_out : Outport  Port=2  VectorParamsAs1DForOutWhenUnconnected=off
  u_out : Outport  Port=3  VectorParamsAs1DForOutWhenUnconnected=off
  v_out : Outport  Port=4  VectorParamsAs1DForOutWhenUnconnected=off
  validOut : Outport  Port=5  VectorParamsAs1DForOutWhenUnconnected=off
  ready : Outport  Port=6  VectorParamsAs1DForOutWhenUnconnected=off
  wires:
  Delay13/1 -> ready/1
  Delay12/1 -> Delay3/1
  Delay10/1 -> MATLAB Function/5(iteration)
  Delay9/1 -> Switch3/2, Switch2/2, Switch1/2, Switch/2
  Delay8/1 -> Switch3/3, Same Datatype2/2(Reference)
  Delay6/1 -> Switch2/3, Same Datatype3/2(Reference)
  Delay5/1 -> Switch1/3, Same Datatype1/2(Reference)
  Delay4/1 -> Switch/3, Same Datatype/2(Reference)
  Same Datatype2/1(DataOut) -> Switch3/1
  Same Datatype3/1(DataOut) -> Switch2/1
  Same Datatype1/1(DataOut) -> Switch1/1
  Same Datatype/1(DataOut) -> Switch/1
  v/1 -> Delay8/1
  u/1 -> Delay6/1
  y/1 -> Delay5/1
  x/1 -> Delay4/1
  CORDIC Counter/1(count_is_positive) -> Delay9/1
  Switch3/1 -> MATLAB Function/4(v)
  Switch2/1 -> MATLAB Function/3(u)
  Switch1/1 -> MATLAB Function/2(y)
  Switch/1 -> MATLAB Function/1(x)
  CORDIC Counter/4(ready) -> Delay13/1
  CORDIC Counter/3(last) -> Delay12/1
  CORDIC Counter/2(count) -> Delay10/1
  validIn/1 -> CORDIC Counter/1(validIn)
  Delay3/1 -> validOut/1
  Delay7/1 -> u_out/1, Same Datatype3/1(Data)
  MATLAB Function/4(v_out) -> Delay11/1
  MATLAB Function/3(u_out) -> Delay7/1
  MATLAB Function/2(y_out) -> Delay2/1
  MATLAB Function/1(x_out) -> Delay1/1
  Delay11/1 -> v_out/1, Same Datatype2/1(Data)
  Delay2/1 -> y_out/1, Same Datatype1/1(Data)
  Delay1/1 -> x_out/1, Same Datatype/1(Data)

== system MVDR_example_hdl_4x4_systolic/MVDR HDL/Compute Weight Vector/Matrix Left Divide/CORDIC/4x4 Complex CORDIC Matrix Left Divide/Q'B, R 4x4 Complex CORDIC Systolic Array/Leading Complex Row Rotation/Rotate first element to real ==
  x : Inport
  u : Inport  Port=2
  validIn : Inport  Port=3
  Complex to Real-Imag : ComplexToRealImag
  Complex to Real-Imag1 : ComplexToRealImag
  Delay{4..7,9..10,15} (7 alike) : Delay  DelayLength=1
  Force imaginary part to exactly zero : MATLAB Function  TreatAsAtomicUnit=on
  Inverse CORDIC Gain1 : Subsystem  TreatAsAtomicUnit=on  mask{NumberOfCORDICIterations=NumberOfCORDICIterations}
      mask prompts: NumberOfCORDICIterations "Number of CORDIC Iterations"
      mask Display: disp('1/An')
  Inverse CORDIC Gain2 : Subsystem  TreatAsAtomicUnit=on  mask{NumberOfCORDICIterations=NumberOfCORDICIterations}
      mask prompts: NumberOfCORDICIterations "Number of CORDIC Iterations"
      mask Display: disp('1/An')
  Inverse CORDIC Gain3 : Subsystem  TreatAsAtomicUnit=on  mask{NumberOfCORDICIterations=NumberOfCORDICIterations}
      mask prompts: NumberOfCORDICIterations "Number of CORDIC Iterations"
      mask Display: disp('1/An')
  Inverse CORDIC Gain4 : Subsystem  TreatAsAtomicUnit=on  mask{NumberOfCORDICIterations=NumberOfCORDICIterations}
      mask prompts: NumberOfCORDICIterations "Number of CORDIC Iterations"
      mask Display: disp('1/An')
  "Q'B, R Row Rotations - Real" : Subsystem  TreatAsAtomicUnit=on  mask{NumberOfCORDICIterations=NumberOfCORDICIterations}
      mask prompts: NumberOfCORDICIterations "Number of CORDIC Iterations"
  QR 3rd and 4th Quadrant Compensation : MATLAB Function  TreatAsAtomicUnit=on
  Real-Imag to Complex : RealImagToComplex
  Real-Imag to Complex1 : RealImagToComplex
  State Control : StateControl  StateControl=Synchronous
  Unit Delay Enabled Synchronous{,1..3} (4 alike) : hdlsllib/Discrete/Unit Delay Enabled Synchronous  InitialCondition=0.0  SampleTime=-1
      settings: SourceProductBaseCode=SL
  ValidIn to Ready Logic with Delay : Subsystem
  x' : Outport  VectorParamsAs1DForOutWhenUnconnected=off
  u' : Outport  Port=2  VectorParamsAs1DForOutWhenUnconnected=off
  validOut : Outport  Port=3  VectorParamsAs1DForOutWhenUnconnected=off
  ready : Outport  Port=4  VectorParamsAs1DForOutWhenUnconnected=off
  wires:
  QR 3rd and 4th Quadrant Compensation/1(x_out) -> Delay4/1
  QR 3rd and 4th Quadrant Compensation/3(u_out) -> Delay6/1
  QR 3rd and 4th Quadrant Compensation/2(y_out) -> Delay5/1
  QR 3rd and 4th Quadrant Compensation/4(v_out) -> Delay7/1
  Complex to Real-Imag/1 -> QR 3rd and 4th Quadrant Compensation/1(x)
  Complex to Real-Imag/2 -> QR 3rd and 4th Quadrant Compensation/2(y)
  Complex to Real-Imag1/1 -> QR 3rd and 4th Quadrant Compensation/3(u)
  Complex to Real-Imag1/2 -> QR 3rd and 4th Quadrant Compensation/4(v)
  Delay4/1 -> "Q'B, R Row Rotations - Real"/1(x)
  Delay5/1 -> "Q'B, R Row Rotations - Real"/2(y)
  Delay6/1 -> "Q'B, R Row Rotations - Real"/3(u)
  Delay7/1 -> "Q'B, R Row Rotations - Real"/4(v)
  "Q'B, R Row Rotations - Real"/1(x_out) -> Inverse CORDIC Gain4/1(In1)
  "Q'B, R Row Rotations - Real"/3(u_out) -> Inverse CORDIC Gain2/1(In1)
  "Q'B, R Row Rotations - Real"/4(v_out) -> Inverse CORDIC Gain3/1(In1)
  x/1 -> Unit Delay Enabled Synchronous1/1
  u/1 -> Unit Delay Enabled Synchronous/1
  "Q'B, R Row Rotations - Real"/2(y_out) -> Inverse CORDIC Gain1/1(In1)
  Force imaginary part to exactly zero/1(y) -> Real-Imag to Complex/2
  Delay9/1 -> ValidIn to Ready Logic with Delay/3(validIn), Delay10/1
  validIn/1 -> Unit Delay Enabled Synchronous/2, Unit Delay Enabled Synchronous1/2, Delay9/1
  Delay10/1 -> ValidIn to Ready Logic with Delay/2(validIn * z^-1), "Q'B, R Row Rotations - Real"/5(validIn)
  Inverse CORDIC Gain4/1(Out1) -> Real-Imag to Complex/1
  Inverse CORDIC Gain1/1(Out1) -> Force imaginary part to exactly zero/1(u)
  Inverse CORDIC Gain2/1(Out1) -> Real-Imag to Complex1/1
  Inverse CORDIC Gain3/1(Out1) -> Real-Imag to Complex1/2
  "Q'B, R Row Rotations - Real"/5(validOut) -> Unit Delay Enabled Synchronous2/2, Unit Delay Enabled Synchronous3/2, Delay15/1
  Delay15/1 -> validOut/1
  ValidIn to Ready Logic with Delay/1(readyOut) -> ready/1
  "Q'B, R Row Rotations - Real"/6(ready) -> ValidIn to Ready Logic with Delay/1(readyIn)
  Unit Delay Enabled Synchronous/1 -> Complex to Real-Imag1/1
  Unit Delay Enabled Synchronous1/1 -> Complex to Real-Imag/1
  Real-Imag to Complex1/1 -> Unit Delay Enabled Synchronous2/1
  Unit Delay Enabled Synchronous2/1 -> u'/1
  Real-Imag to Complex/1 -> Unit Delay Enabled Synchronous3/1
  Unit Delay Enabled Synchronous3/1 -> x'/1
